simulink model "originalProcess"  (R2019a)
settings: Solver=VariableStepAuto  StartTime=0.0  StopTime=100  RelTol=1e-3
settings Model: Creator=Administrator  LastModifiedBy=Administrator

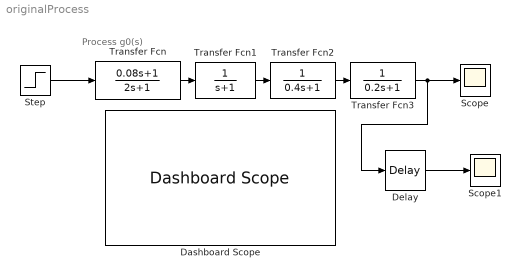
== system originalProcess ==
  note: Process g0(s)
  Dashboard Scope : DashboardScope
  Delay : TransportDelay  DelayTime=3
  Scope : Scope
  Scope1 : Scope
  Step : Step  SampleTime=0
  Transfer Fcn : TransferFcn  Numerator=[0.08 1]  Denominator=[2 1]
  Transfer Fcn1 : TransferFcn  Denominator=[1 1]
  Transfer Fcn2 : TransferFcn  Denominator=[0.4 1]
  Transfer Fcn3 : TransferFcn  Denominator=[0.2 1]
  wires:
  Transfer Fcn/1 -> Transfer Fcn1/1
  Transfer Fcn1/1 -> Transfer Fcn2/1
  Transfer Fcn2/1 -> Transfer Fcn3/1
  Transfer Fcn3/1 -> Delay/1, Scope/1
  Delay/1 -> Scope1/1
  Step/1 -> Transfer Fcn/1
